simulink model "modelFree"  (R2022b)
settings: Solver=ode45  StartTime=0.0  StopTime=10  FixedStep=0.05  RelTol=1e-10
settings Model: Creator=pedram  LastModifiedBy=alish
settings DataIOCC: SaveOutput=off

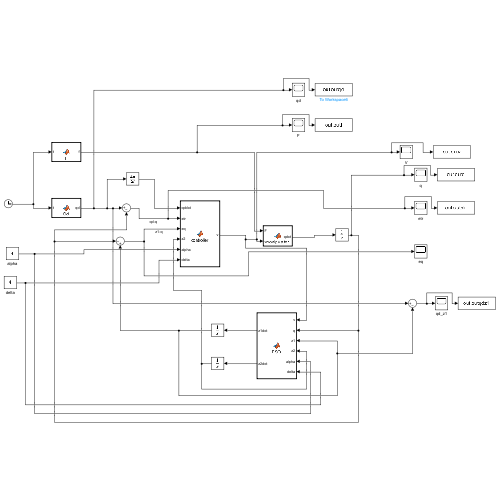
[thumbnail: Simulink's stored preview of the top-level diagram]
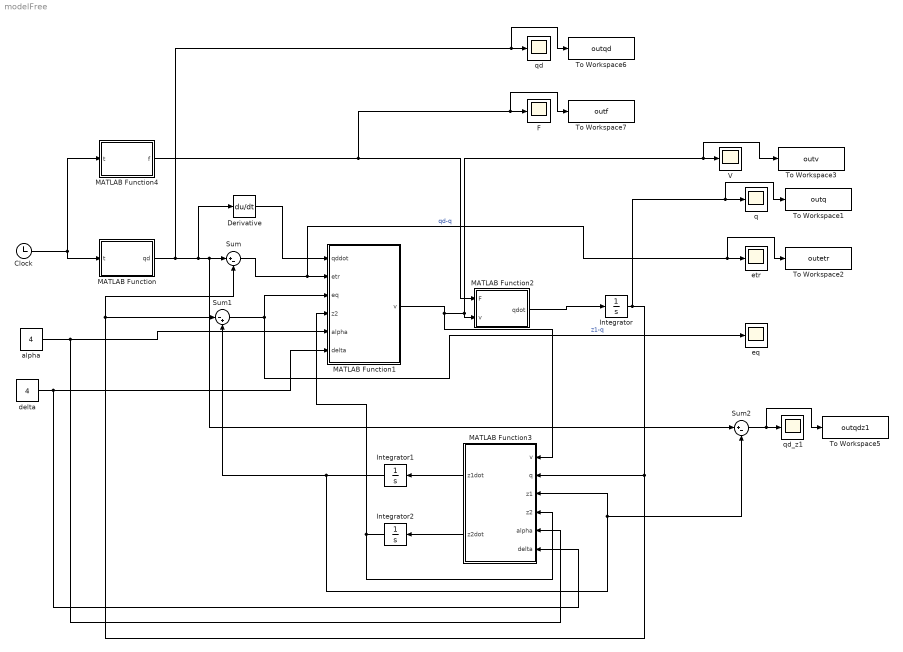
== system modelFree ==
  Clock : Clock
  Derivative : Derivative
  F : Scope
  Integrator : Integrator
  Integrator1 : Integrator
  Integrator2 : Integrator
  MATLAB Function : MATLAB Function  TreatAsAtomicUnit=on
  MATLAB Function1 : MATLAB Function  TreatAsAtomicUnit=on
  MATLAB Function2 : MATLAB Function  TreatAsAtomicUnit=on
  MATLAB Function3 : MATLAB Function  TreatAsAtomicUnit=on
  MATLAB Function4 : MATLAB Function  TreatAsAtomicUnit=on
  Sum : Sum  Inputs=|+-
  Sum1 : Sum  Inputs=|-+
  Sum2 : Sum  Inputs=|+-
  To Workspace1 : ToWorkspace  VariableName=outq  SampleTime=-1
      settings: Save2DSignal=2-D array (concatenate along first dimension)
  To Workspace2 : ToWorkspace  VariableName=outetr  SampleTime=-1
      settings: Save2DSignal=2-D array (concatenate along first dimension)
  To Workspace3 : ToWorkspace  VariableName=outv  SampleTime=-1
      settings: Save2DSignal=2-D array (concatenate along first dimension)
  To Workspace5 : ToWorkspace  VariableName=outqdz1  SampleTime=-1
      settings: Save2DSignal=2-D array (concatenate along first dimension)
  To Workspace6 : ToWorkspace  VariableName=outqd  SampleTime=-1
      settings: Save2DSignal=2-D array (concatenate along first dimension)
  To Workspace7 : ToWorkspace  VariableName=outf  SampleTime=-1
      settings: Save2DSignal=2-D array (concatenate along first dimension)
  V : Scope
  alpha : Constant  Value=4
  delta : Constant  Value=4
  eq : Scope
  etr : Scope
  q : Scope
  qd : Scope
  qd_z1 : Scope
  wires:
  Sum2/1 -> qd_z1/1, To Workspace5/1
  MATLAB Function1/1(v) -> MATLAB Function3/1(v), To Workspace3/1, V/1, MATLAB Function2/2(v)
  Derivative/1 -> MATLAB Function1/1(qddot)
  Integrator1/1 -> Sum1/2, Sum2/2, MATLAB Function3/3(z1)
  Integrator2/1 -> MATLAB Function1/4(z2), MATLAB Function3/4(z2)
  Sum1/1 -> eq/1, MATLAB Function1/3(eq)  "z1-q"
  Clock/1 -> MATLAB Function4/1(t), MATLAB Function/1(t)
  MATLAB Function3/2(z2dot) -> Integrator2/1
  MATLAB Function2/1(qdot) -> Integrator/1
  MATLAB Function/1(qd) -> To Workspace6/1, qd/1, Derivative/1, Sum2/1, Sum/1
  Integrator/1 -> To Workspace1/1, q/1, Sum1/1, Sum/2, MATLAB Function3/2(q)
  Sum/1 -> To Workspace2/1, etr/1, MATLAB Function1/2(etr)  "qd-q"
  MATLAB Function3/1(z1dot) -> Integrator1/1
  MATLAB Function4/1(f) -> To Workspace7/1, F/1, MATLAB Function2/1(F)
  alpha/1 -> MATLAB Function3/5(alpha), MATLAB Function1/5(alpha)
  delta/1 -> MATLAB Function3/6(delta), MATLAB Function1/6(delta)

== matlab function modelFree/MATLAB Function1 ==
  data: qddot input; v output; etr input; eq input; z2 input; alpha input; delta input
function v = controller(qddot,etr,eq,z2,alpha,delta)
% delta=0.8;
% alpha=0.8;

beta1=diag([50,50,30]);
Kp=diag([50,200,100]);
v=zeros(3,1);
    if norm(eq,2)<=delta
    v=qddot+Kp*(etr-eq)+beta1*(eq./delta^(1-alpha))-z2;
    elseif norm(eq,2)>delta
    v=qddot+Kp*(etr-eq)+beta1*(norm(eq,2)^alpha.*sign(eq))-z2;
    end
    for i=1:3
        if v(i)>40
        v(i)=40;
    elseif v(i)<-40
        v(i)=-40;
        end
    end

== matlab function modelFree/MATLAB Function ==
  data: t input; qd output
function qd = Qd(t)

qd = [1-cos(0.1*pi*t);1-cos(0.1*pi*t);1-cos(0.1*pi*t)];

== matlab function modelFree/MATLAB Function2 ==
  data: F input; v input; qdot output
function qdot = manipulator(F,v)

qdot=v+F;

== matlab function modelFree/MATLAB Function3 ==
  data: v input; q input; z1dot output; z1 input; z2 input; z2dot output; alpha input; delta input
function [z1dot,z2dot]= ESO(v,q,z1,z2,alpha,delta)
% delta=0.8;
% alpha=0.8;
eq=z1-q;

beta1=diag([50,50,30]);
beta2=diag([50,50,40]);

c1=beta1./(delta^(1-alpha));
z1dot=zeros(3,1);
z2dot=zeros(3,1);

if norm(eq,2)<=delta
    z1dot=z2-c1*eq+v;
    z2dot=-c1*eq;
%     z1dot = z2 - beta1 * eq ./ delta^(1-alpha) + v;
%     z2dot = -beta2 * eq ./delta^(1-alpha);
elseif norm(eq,2)>delta
    z1dot=z2-beta1*(norm(eq,2)^alpha*sign(eq))+v;
    z2dot=-beta2*(norm(eq,2)^(2*alpha-1)*sign(eq));
end

== matlab function modelFree/MATLAB Function4 ==
  data: t input; f output
  function f = F(t)

f=zeros(3,1);
if t<4
    f=zeros(3,1);
elseif t>=4 && t<7
    f=(15).*[1;1;1];
else
    f=(15+10*sin(pi*t)).*[1;1;1];
end
